simulink model "ventilator"  (R2021b)
settings: Solver=VariableStepAuto  StartTime=0.0  StopTime=15  MaxStep=0.01  RelTol=1e-3
values from neighbouring files (symbols this model uses):
  Kd = PID(3)    [simulate.m]
  Ki = PID(2)    [simulate.m]
  Kp = PID(1)    [simulate.m]
libraries: slpidlib x2
settings Model: Creator=victormu98  LastModifiedBy=victormu98

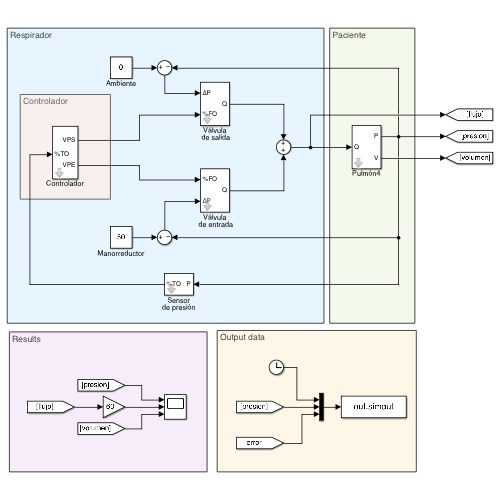
[thumbnail: Simulink's stored preview of the top-level diagram]
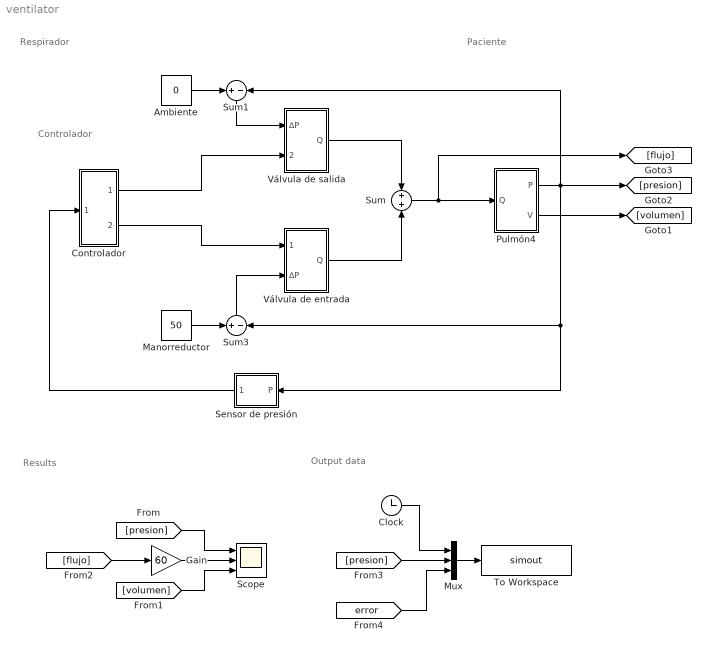
== system ventilator ==
  note: Output data
  note: Results
  note: Controlador
  note: Paciente
  note: Respirador
  Ambiente : Constant  Value=0
  Clock : Clock
  Controlador : Subsystem  mask{SP=30, PEEP=10, FR=12, IE=2/3}
      mask prompts: SP "Consigna (mbar)"; PEEP "PEEP (mbar)"; FR "Frecuencia respiratoria (resp/min)"; IE "I:E"
      mask DialogControl Container7 Prompt: Parámetros
  Gain : Gain  Gain=60
  Manorreductor : Constant  Value=50
  Mux : Mux  Inputs=3
  Pulmón4 : Subsystem  mask{R=20, C1=0.023, C2=0.1}
  Scope : Scope  NumInputPorts=3
  Sensor de presión : Subsystem  mask{Ks=0.01}
      mask prompts: Ks "Ganancia"
  Sum : Sum
  Sum1 : Sum  Inputs=+|-
  Sum3 : Sum  Inputs=+|-
  To Workspace : ToWorkspace  VariableName=simout  SaveFormat=Timeseries  SampleTime=-1
  Válvula de entrada : Subsystem  mask{D=0.004, tau=0.075}
      mask prompts: D "Diámetro"; tau "Constante de tiempo"
  Válvula de salida : Subsystem  mask{D=0.004, tau=0.075}
      mask prompts: D "Diámetro"; tau "Constante de tiempo"
  wires:
  Manorreductor/1 -> Sum3/1
  Pulmón4/2(V) -> [volumen]
  Válvula de salida/1(Q) -> Sum/1
  Sum1/1 -> Válvula de salida/1(∆P)
  Válvula de entrada/1(Q) -> Sum/2
  Ambiente/1 -> Sum1/1
  Sum3/1 -> Válvula de entrada/2(∆P)
  Sensor de presión/1(%TO) -> Controlador/1(%TO)
  Sum/1 -> [flujo], Pulmón4/1(Q)
  [flujo] -> Gain/1
  Pulmón4/1(P) -> Sum1/2, [presion], Sensor de presión/1(P), Sum3/2
  Gain/1 -> Scope/2
  [presion] -> Scope/1
  [volumen] -> Scope/3
  Controlador/1(VPS) -> Válvula de salida/2(%FO)
  Controlador/2(VPE) -> Válvula de entrada/1(%FO)
  Mux/1 -> To Workspace/1
  Clock/1 -> Mux/1
  [presion] -> Mux/2
  [error] -> Mux/3

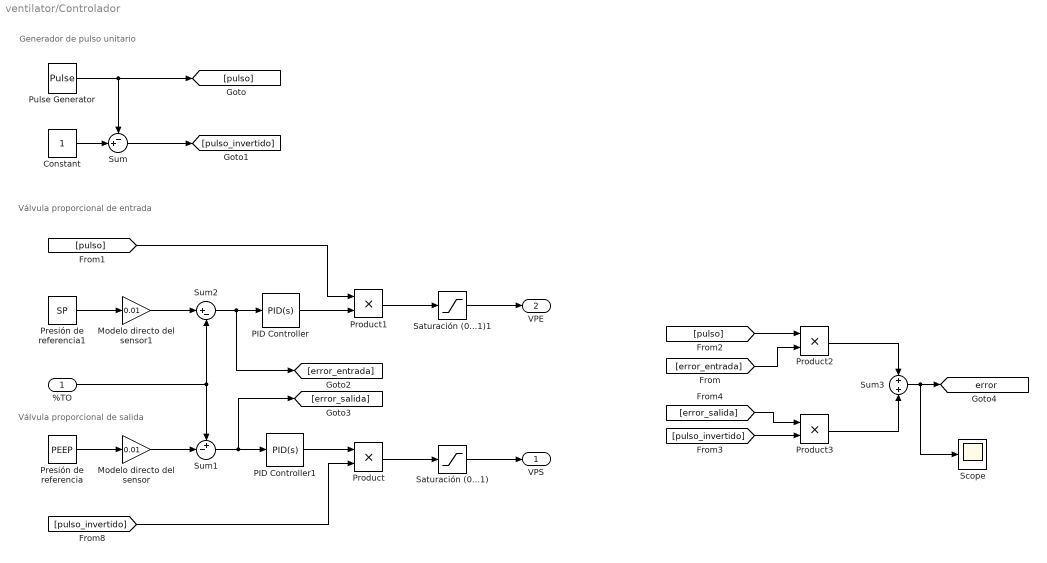
== system ventilator/Controlador ==
  note: Generador de pulso unitario
  note: Válvula proporcional de salida
  note: Válvula proporcional de entrada
  %TO : Inport
  Constant : Constant
  Modelo directo del sensor : Gain  Gain=0.01
  Modelo directo del sensor1 : Gain  Gain=0.01
  PID Controller : slpidlib/PID Controller  Controller=PID  Form=Parallel  TimeDomain=Continuous-time  UseExternalTs=off  SampleTime=-1  IntegratorMethod=Forward Euler  FilterMethod=Forward Euler  ControllerParametersSource=internal  P=Kp  I=Ki  D=Kd  UseFilter=on  N=100  TunerSelectOption=Transfer Function Based (PID Tuner App)  InitialConditionSource=internal  InitialConditionForIntegrator=0  InitialConditionForFilter=0  DifferentiatorICPrevScaledInput=0  ExternalReset=none  TrackingMode=off  Kt=1  LimitOutput=off  SatLimitsSource=internal  UpperSaturationLimit=inf  LowerSaturationLimit=-inf  LinearizeAsGain=on  AntiWindupMode=none  Kb=1  POutMin=[]  POutMax=[]  IOutMin=[]  IOutMax=[]  DOutMin=[]  DOutMax=[]  NOutMin=[]  NOutMax=[]  SumOutMin=[]  SumOutMax=[]  SaturationOutMin=[]  SaturationOutMax=[]  PParamMin=[]  PParamMax=[]  IParamMin=[]  IParamMax=[]  DParamMin=[]  DParamMax=[]  NParamMin=[]  NParamMax=[]  KbParamMin=[]  KbParamMax=[]  KtParamMin=[]  KtParamMax=[]  KbOutMin=[]  KbOutMax=[]  KtOutMin=[]  KtOutMax=[]  IntegratorOutMin=[]  IntegratorOutMax=[]  FilterOutMin=[]  FilterOutMax=[]  SumI1OutMin=[]  SumI1OutMax=[]  SumI2OutMin=[]  SumI2OutMax=[]  SumI3OutMin=[]  SumI3OutMax=[]  SumI4OutMin=[]  SumI4OutMax=[]  SumDOutMin=[]  SumDOutMax=[]  DifferentiatorOutMin=[]  DifferentiatorOutMax=[]  FilterDiffOutCoefMin=[]  FilterDiffOutCoefMax=[]  ReciprocalOutMin=[]  ReciprocalOutMax=[]  SumDenOutMin=[]  SumDenOutMax=[]  SumNumOutMin=[]  SumNumOutMax=[]  DivideOutMin=[]  DivideOutMax=[]  UdiffTsProdOutMin=[]  UdiffTsProdOutMax=[]  NTsProdOutMin=[]  NTsProdOutMax=[]  UintegralTsProdOutMin=[]  UintegralTsProdOutMax=[]  UngainTsProdOutMin=[]  UngainTsProdOutMax=[]  IntegratorContinuousStateAttributes=''  IntegratorStateMustResolveToSignalObject=off  IntegratorRTWStateStorageClass=Auto  FilterContinuousStateAttributes=''  FilterStateMustResolveToSignalObject=off  FilterRTWStateStorageClass=Auto  ParallelPVariant=InternalParameters  IdealPVariant=Disabled  IVariant=InternalParameters  DVariant=InternalParameters  IntegratorVariant=Continuous  SatVariant=Disabled  AWVariant=Passthrough  PCopyVariant=Disabled  TRVariant=Disabled  FdbkBlocksVariant=Forward  IdealPFdbkVariant=Disabled  SatFdbkVariant=Disabled  DerivativeFilterVariant=ContFilter  NVariant=InternalParameters  NCopyVariant=Disabled  FilterICVariant=InternalICsFilter  IntegratorICVariant=InternalICs  ExternalResetVariant=Disabled  TRSumVariant=Passthrough  SumFdbkVariant=Disabled  SumVariant=Sum_PID  TsampFilterVariant=InternalTs  TsampNgainVariant=Passthrough  TsampIntegralVariant=Passthrough  ExternalSaturationOutDataTypeStr=Inherit: Same as second input
  PID Controller1 : slpidlib/PID Controller  Controller=PID  Form=Parallel  TimeDomain=Continuous-time  UseExternalTs=off  SampleTime=-1  IntegratorMethod=Forward Euler  FilterMethod=Forward Euler  ControllerParametersSource=internal  P=Kp  I=Ki  D=Kd  UseFilter=on  N=100  TunerSelectOption=Transfer Function Based (PID Tuner App)  InitialConditionSource=internal  InitialConditionForIntegrator=0  InitialConditionForFilter=0  DifferentiatorICPrevScaledInput=0  ExternalReset=none  TrackingMode=off  Kt=1  LimitOutput=off  SatLimitsSource=internal  UpperSaturationLimit=inf  LowerSaturationLimit=-inf  LinearizeAsGain=on  AntiWindupMode=none  Kb=1  POutMin=[]  POutMax=[]  IOutMin=[]  IOutMax=[]  DOutMin=[]  DOutMax=[]  NOutMin=[]  NOutMax=[]  SumOutMin=[]  SumOutMax=[]  SaturationOutMin=[]  SaturationOutMax=[]  PParamMin=[]  PParamMax=[]  IParamMin=[]  IParamMax=[]  DParamMin=[]  DParamMax=[]  NParamMin=[]  NParamMax=[]  KbParamMin=[]  KbParamMax=[]  KtParamMin=[]  KtParamMax=[]  KbOutMin=[]  KbOutMax=[]  KtOutMin=[]  KtOutMax=[]  IntegratorOutMin=[]  IntegratorOutMax=[]  FilterOutMin=[]  FilterOutMax=[]  SumI1OutMin=[]  SumI1OutMax=[]  SumI2OutMin=[]  SumI2OutMax=[]  SumI3OutMin=[]  SumI3OutMax=[]  SumI4OutMin=[]  SumI4OutMax=[]  SumDOutMin=[]  SumDOutMax=[]  DifferentiatorOutMin=[]  DifferentiatorOutMax=[]  FilterDiffOutCoefMin=[]  FilterDiffOutCoefMax=[]  ReciprocalOutMin=[]  ReciprocalOutMax=[]  SumDenOutMin=[]  SumDenOutMax=[]  SumNumOutMin=[]  SumNumOutMax=[]  DivideOutMin=[]  DivideOutMax=[]  UdiffTsProdOutMin=[]  UdiffTsProdOutMax=[]  NTsProdOutMin=[]  NTsProdOutMax=[]  UintegralTsProdOutMin=[]  UintegralTsProdOutMax=[]  UngainTsProdOutMin=[]  UngainTsProdOutMax=[]  IntegratorContinuousStateAttributes=''  IntegratorStateMustResolveToSignalObject=off  IntegratorRTWStateStorageClass=Auto  FilterContinuousStateAttributes=''  FilterStateMustResolveToSignalObject=off  FilterRTWStateStorageClass=Auto  ParallelPVariant=InternalParameters  IdealPVariant=Disabled  IVariant=InternalParameters  DVariant=InternalParameters  IntegratorVariant=Continuous  SatVariant=Disabled  AWVariant=Passthrough  PCopyVariant=Disabled  TRVariant=Disabled  FdbkBlocksVariant=Forward  IdealPFdbkVariant=Disabled  SatFdbkVariant=Disabled  DerivativeFilterVariant=ContFilter  NVariant=InternalParameters  NCopyVariant=Disabled  FilterICVariant=InternalICsFilter  IntegratorICVariant=InternalICs  ExternalResetVariant=Disabled  TRSumVariant=Passthrough  SumFdbkVariant=Disabled  SumVariant=Sum_PID  TsampFilterVariant=InternalTs  TsampNgainVariant=Passthrough  TsampIntegralVariant=Passthrough  ExternalSaturationOutDataTypeStr=Inherit: Same as second input
  Presión de referencia : Constant  Value=PEEP
  Presión de referencia1 : Constant  Value=SP
  Product{,1..3} (4 alike) : Product
  Pulse Generator : DiscretePulseGenerator  PulseType=Time based  Period=60/FR  PulseWidth=IE/(IE+1)*100
  Saturación (0...1) : Saturate  UpperLimit=1  LowerLimit=0
  Saturación (0...1)1 : Saturate  UpperLimit=1  LowerLimit=0
  Scope : Scope
  Sum : Sum  Inputs=-+|
  Sum1 : Sum  Inputs=+-|
  Sum2 : Sum  Inputs=|+-
  Sum3 : Sum  Inputs=+|+
  VPS : Outport
  VPE : Outport  Port=2
  tag scope: error=global
  wires:
  Sum/1 -> [pulso_invertido]
  Pulse Generator/1 -> [pulso], Sum/1
  Constant/1 -> Sum/2
  %TO/1 -> Sum1/1, Sum2/2
  Presión de referencia/1 -> Modelo directo del sensor/1
  Product/1 -> Saturación (0...1)/1
  Saturación (0...1)/1 -> VPS/1
  PID Controller1/1 -> Product/1
  Modelo directo del sensor/1 -> Sum1/2
  [pulso_invertido] -> Product/2
  Sum2/1 -> [error_entrada], PID Controller/1
  Saturación (0...1)1/1 -> VPE/1
  Product1/1 -> Saturación (0...1)1/1
  Presión de referencia1/1 -> Modelo directo del sensor1/1
  [pulso] -> Product1/1
  PID Controller/1 -> Product1/2
  Modelo directo del sensor1/1 -> Sum2/1
  Sum1/1 -> [error_salida], PID Controller1/1
  [pulso] -> Product2/1
  [pulso_invertido] -> Product3/2
  [error_salida] -> Product3/1
  [error_entrada] -> Product2/2
  Product3/1 -> Sum3/2
  Product2/1 -> Sum3/1
  Sum3/1 -> Scope/1, [error]

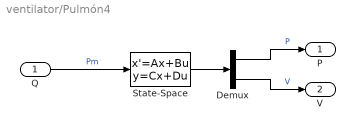
== system ventilator/Pulmón4 ==
  Q : Inport
  Demux : Demux  Outputs=2
  State-Space : StateSpace  A=[-1/(R*C2) 1/(R*C1*C2) ; 0 0]  B=[(C1+C2)/(C1*C2) ; 1]  C=[1 0 ; 0 1]  D=[0 ; 0]  InitialCondition=0
  P : Outport
  V : Outport  Port=2
  wires:
  Q/1 -> State-Space/1  "Pm"
  State-Space/1 -> Demux/1
  Demux/1 -> P/1  "P"
  Demux/2 -> V/1  "V"

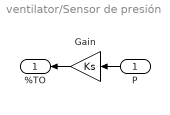
== system ventilator/Sensor de presión ==
  P : Inport
  Gain : Gain  Gain=Ks
  %TO : Outport
  wires:
  Gain/1 -> %TO/1
  P/1 -> Gain/1

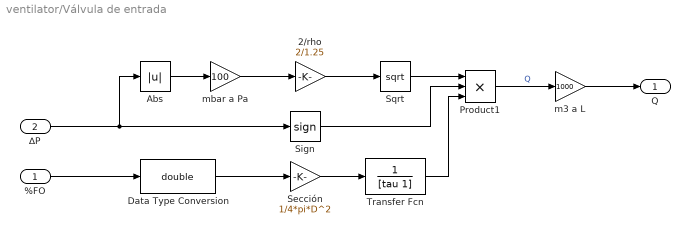
== system ventilator/Válvula de entrada ==
  %FO : Inport
  ∆P : Inport  Port=2
  2/rho : Gain  Gain=2/1.25
  Abs : Abs
  Data Type Conversion : DataTypeConversion  OutDataTypeStr=double
  Product1 : Product  Inputs=3
  Sección : Gain  Gain=1/4*pi*D^2
  Sign : Signum
  Sqrt : Sqrt  SaturateOnIntegerOverflow=on
  Transfer Fcn : TransferFcn  Denominator=[tau 1]
  m3 a L : Gain  Gain=1000
  mbar a Pa : Gain  Gain=100
  Q : Outport
  wires:
  Transfer Fcn/1 -> Product1/3
  Data Type Conversion/1 -> Sección/1
  %FO/1 -> Data Type Conversion/1
  Sección/1 -> Transfer Fcn/1
  mbar a Pa/1 -> 2/rho/1
  Sign/1 -> Product1/2
  ∆P/1 -> Abs/1, Sign/1
  Abs/1 -> mbar a Pa/1
  Product1/1 -> m3 a L/1  "Q"
  Sqrt/1 -> Product1/1
  2/rho/1 -> Sqrt/1
  m3 a L/1 -> Q/1

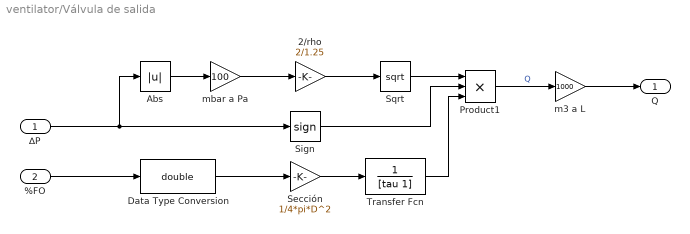
== system ventilator/Válvula de salida ==
  ∆P : Inport
  %FO : Inport  Port=2
  2/rho : Gain  Gain=2/1.25
  Abs : Abs
  Data Type Conversion : DataTypeConversion  OutDataTypeStr=double
  Product1 : Product  Inputs=3
  Sección : Gain  Gain=1/4*pi*D^2
  Sign : Signum
  Sqrt : Sqrt  SaturateOnIntegerOverflow=on
  Transfer Fcn : TransferFcn  Denominator=[tau 1]
  m3 a L : Gain  Gain=1000
  mbar a Pa : Gain  Gain=100
  Q : Outport
  wires:
  m3 a L/1 -> Q/1
  2/rho/1 -> Sqrt/1
  Sqrt/1 -> Product1/1
  Product1/1 -> m3 a L/1  "Q"
  Abs/1 -> mbar a Pa/1
  ∆P/1 -> Sign/1, Abs/1
  Sign/1 -> Product1/2
  mbar a Pa/1 -> 2/rho/1
  Sección/1 -> Transfer Fcn/1
  %FO/1 -> Data Type Conversion/1
  Data Type Conversion/1 -> Sección/1
  Transfer Fcn/1 -> Product1/3
